simulink library "mat_4x4"  (R2020b)
settings: Solver=VariableStepAuto  StartTime=0.0  StopTime=10.0  RelTol=1e-3
settings Model: Creator=whitehole  LastModifiedBy=whitehole

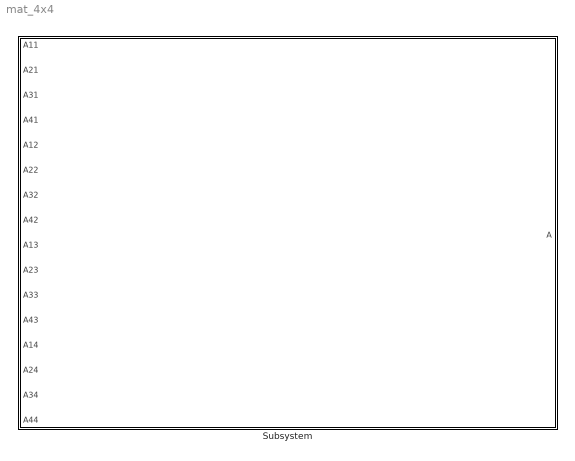
== system mat_4x4 ==
  Subsystem : Subsystem

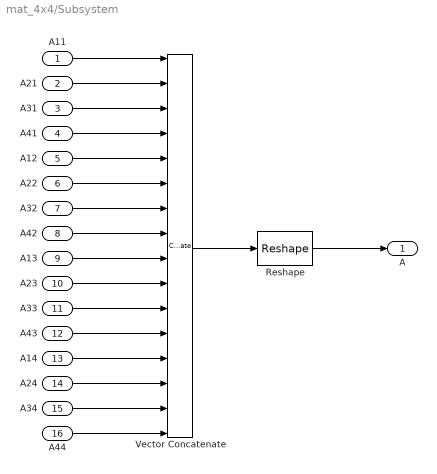
== system mat_4x4/Subsystem ==
  A11 : Inport
  A21 : Inport  Port=2
  A31 : Inport  Port=3
  A41 : Inport  Port=4
  A12 : Inport  Port=5
  A22 : Inport  Port=6
  A32 : Inport  Port=7
  A42 : Inport  Port=8
  A13 : Inport  Port=9
  A23 : Inport  Port=10
  A33 : Inport  Port=11
  A43 : Inport  Port=12
  A14 : Inport  Port=13
  A24 : Inport  Port=14
  A34 : Inport  Port=15
  A44 : Inport  Port=16
  Reshape : Reshape  OutputDimensionality=Customize  OutputDimensions=[4,4]
  Vector Concatenate : Concatenate  NumInputs=16
  A : Outport
  wires:
  A34/1 -> Vector Concatenate/15
  A33/1 -> Vector Concatenate/11
  A13/1 -> Vector Concatenate/9
  A44/1 -> Vector Concatenate/16
  A23/1 -> Vector Concatenate/10
  A12/1 -> Vector Concatenate/5
  A41/1 -> Vector Concatenate/4
  A43/1 -> Vector Concatenate/12
  Reshape/1 -> A/1
  Vector Concatenate/1 -> Reshape/1
  A22/1 -> Vector Concatenate/6
  A21/1 -> Vector Concatenate/2
  A14/1 -> Vector Concatenate/13
  A42/1 -> Vector Concatenate/8
  A32/1 -> Vector Concatenate/7
  A11/1 -> Vector Concatenate/1
  A31/1 -> Vector Concatenate/3
  A24/1 -> Vector Concatenate/14
